simulink model "ad9361_rx_fastattack"  (R2017b)
settings: Solver=ode23  StartTime=0.0  StopTime=inf  RelTol=1e-3  EnableMultiTasking=on
PreLoadFcn:
  | SampleTime_rx = 6.51041666666666667e-8;
  | 
  | adi9361_preload(bdroot,'rx')
undefined symbols (not defined in the file or in its folder): D, dBval, DCLeak_Matrix, fuzz_val, GainImb_Matrix, IP2_Matrix, IP3_Matrix, magnitude, var
libraries: simrfV2elements x13, dsparch4 x8, dspsrcs4 x8, dspmathops x6, dspmlti4 x5, simulink x5, simrfV2util1 x4, fl_lib x4, simrfV2junction1 x3, simulink_extras x2, dspsigattribs x2, simrfV2sources1 x2
(part 2 of 2)

== system ad9361_rx_fastattack/ADI9361_rx/ADC_RX/ADC_Q/Quantizer1 ==
  u : Inport
  Abs : Abs
  Idealized ADC quantizer : simulink_extras/Additional Discrete/Idealized ADC quantizer  NumberOfConverterBits=3  Vmin=0  Vmax=.8  OutputDataType=double  OutputNegativeValues=off
      settings: SourceProductName=Simulink
  Product : Product
  Saturation : Saturate  UpperLimit=0.41
  Sign : Signum
  y : Outport
  wires:
  u/1 -> Sign/1, Abs/1
  Saturation/1 -> Idealized ADC quantizer/1
  Idealized ADC quantizer/1 -> Product/1
  Sign/1 -> Product/2
  Abs/1 -> Saturation/1
  Product/1 -> y/1

== system ad9361_rx_fastattack/ADI9361_rx/DDC_Filters_RX/Hm1/Hm1 ==
  In : Inport
  Hm1 : dspmlti4/FIR Decimation  FilterSource=Filter object  h=fir1(35,0.4)  D=2  filtStruct=Direct form  FilterObject=ad9361_rx_pars.Hm1_rx  framing=Allow multirate processing  inputOffset=0  outputBufInitCond=0  roundingMode=Floor  overflowMode=off  firstCoeffDataTypeStr=Inherit: Same word length as input  firstCoeffMin=[]  firstCoeffMax=[]  firstCoeffLastDataTypeStr=Inherit: Same word length as input  outputDataTypeStr=Inherit: Same as accumulator  outputMin=[]  outputMax=[]  outputLastDataTypeStr=Inherit: Same as accumulator
  Out : Outport
  wires:
  In/1 -> Hm1/1
  Hm1/1 -> Out/1

== system ad9361_rx_fastattack/ADI9361_rx/DDC_Filters_RX/Hm1/NoFilter ==
  In : Inport
  Out : Outport
  wires:
  In/1 -> Out/1

== system ad9361_rx_fastattack/ADI9361_rx/DDC_Filters_RX/Hm2/Hm2 ==
  In : Inport
  Data Type Conversion3 : DataTypeConversion  OutDataTypeStr=fixdt(1,16,14)  RndMeth=Round
  Hm2 : dspmlti4/FIR Decimation  FilterSource=Filter object  h=fir1(35,0.4)  D=2  filtStruct=Direct form  FilterObject=ad9361_rx_pars.Hm2_rx  framing=Allow multirate processing  inputOffset=0  outputBufInitCond=0  roundingMode=Floor  overflowMode=off  firstCoeffDataTypeStr=Inherit: Same word length as input  firstCoeffMin=[]  firstCoeffMax=[]  firstCoeffLastDataTypeStr=Inherit: Same word length as input  outputDataTypeStr=Inherit: Same as accumulator  outputMin=[]  outputMax=[]  outputLastDataTypeStr=Inherit: Same as accumulator
  Out : Outport
  wires:
  In/1 -> Data Type Conversion3/1
  Hm2/1 -> Out/1
  Data Type Conversion3/1 -> Hm2/1

== system ad9361_rx_fastattack/ADI9361_rx/DDC_Filters_RX/Hm2/NoFilter ==
  In : Inport
  Data Type Conversion3 : DataTypeConversion  OutDataTypeStr=fixdt(1,16,14)  RndMeth=Round
  Out : Outport
  wires:
  In/1 -> Data Type Conversion3/1
  Data Type Conversion3/1 -> Out/1

== system ad9361_rx_fastattack/ADI9361_rx/DDC_Filters_RX/Hm3/Hm3 ==
  In : Inport
  Mh3 : dspmlti4/FIR Decimation  FilterSource=Filter object  h=fir1(35,0.4)  D=2  filtStruct=Direct form  FilterObject=ad9361_rx_pars.Hm3_rx  framing=Allow multirate processing  inputOffset=0  outputBufInitCond=0  roundingMode=Floor  overflowMode=off  firstCoeffDataTypeStr=Inherit: Same word length as input  firstCoeffMin=[]  firstCoeffMax=[]  firstCoeffLastDataTypeStr=Inherit: Same word length as input  outputDataTypeStr=Inherit: Same as accumulator  outputMin=[]  outputMax=[]  outputLastDataTypeStr=Inherit: Same as accumulator
  Out : Outport
  wires:
  In/1 -> Mh3/1
  Mh3/1 -> Out/1

== system ad9361_rx_fastattack/ADI9361_rx/DDC_Filters_RX/Hm3/NoFilter ==
  In : Inport
  Out : Outport
  wires:
  In/1 -> Out/1

== system ad9361_rx_fastattack/ADI9361_rx/DDC_Filters_RX/Hm4/Hm4 ==
  In1 : Inport
  Data Type Conversion : DataTypeConversion  OutDataTypeStr=fixdt(1,4,2)  RndMeth=Round
  Hm1 : dspmlti4/FIR Decimation  FilterSource=Filter object  h=fir1(35,0.4)  D=2  filtStruct=Direct form  FilterObject=ad9361_rx_pars.Hm4_rx  framing=Allow multirate processing  inputOffset=0  outputBufInitCond=0  roundingMode=Floor  overflowMode=off  firstCoeffDataTypeStr=Inherit: Same word length as input  firstCoeffMin=[]  firstCoeffMax=[]  firstCoeffLastDataTypeStr=Inherit: Same word length as input  outputDataTypeStr=Inherit: Same as accumulator  outputMin=[]  outputMax=[]  outputLastDataTypeStr=Inherit: Same as accumulator
  Out1 : Outport
  wires:
  In1/1 -> Data Type Conversion/1
  Hm1/1 -> Out1/1
  Data Type Conversion/1 -> Hm1/1

== system ad9361_rx_fastattack/ADI9361_rx/DDC_Filters_RX/Hm4/NoFilter ==
  In1 : Inport
  Data Type Conversion : DataTypeConversion  OutDataTypeStr=fixdt(1,4,2)  RndMeth=Round
  Out1 : Outport
  wires:
  In1/1 -> Data Type Conversion/1
  Data Type Conversion/1 -> Out1/1

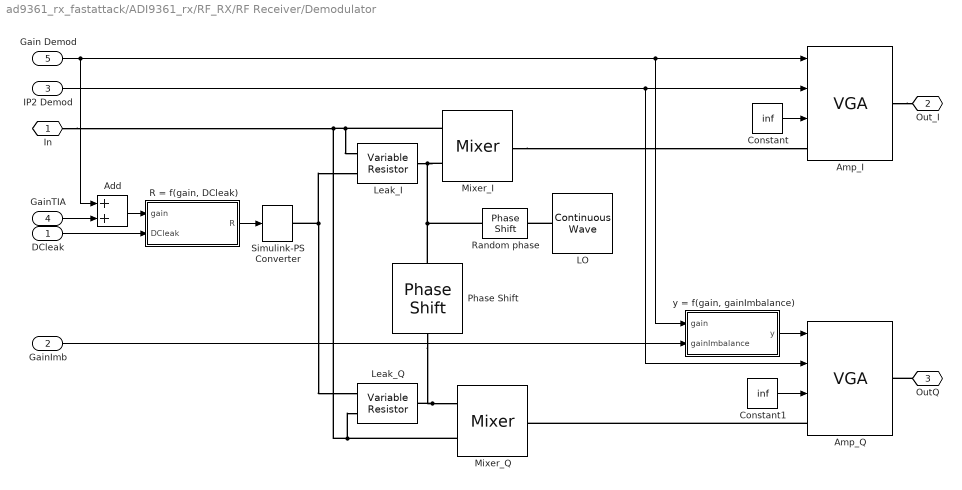
== system ad9361_rx_fastattack/ADI9361_rx/RF_RX/RF Receiver/Demodulator ==
  DCleak : Inport
  GainImb : Inport  Port=2
  IP2 Demod : Inport  Port=3
  GainTIA : Inport  Port=4
  Gain Demod : Inport  Port=5
  Add : Sum
  Amp_I : simrfV2elements/VGA  classname=vga  Zin=100  Zout=100  IO=Input  InternalGrounding=on
      settings: SourceProductName=RF Blockset  SourceProductBaseCode=RB
  Amp_Q : simrfV2elements/VGA  classname=vga  Zin=100  Zout=100  IO=Input  InternalGrounding=on
      settings: SourceProductName=RF Blockset  SourceProductBaseCode=RB
  Constant : Constant  Value=inf
  Constant1 : Constant  Value=inf
  LO : simrfV2sources1/Continuous Wave  CWSourceType=Ideal voltage  Z0=0  IVoltage=1/sqrt(2) V  ICurrent=0 A  MagPower=1 W  QVoltage=0 V  QCurrent=0 A  AnglePower=0  CarrierFreq=RF Hz  InternalGrounding=on
      settings: SourceProductName=RF Blockset  SourceProductBaseCode=RB
  Leak_I : fl_lib/Electrical/Electrical Elements/Variable Resistor  Rmin=0 Ohm  i_specify=off  i_priority=High  i=0 A  v_specify=off  v_priority=High  v=0 V
  Leak_Q : fl_lib/Electrical/Electrical Elements/Variable Resistor  Rmin=0 Ohm  i_specify=off  i_priority=High  i=0 A  v_specify=off  v_priority=High  v=0 V
  Mixer_I : simrfV2elements/Mixer  classname=mixer  Source_linear_gain=Available power gain  linear_gain=0 dB  Zin=100  Zout=100  ZLO=inf  Source_Poly=Even and odd order  Poly_Coeffs=[0 1]  IPType=Output  IP2=Inf dBm  IP3=Inf dBm  P1dB=Inf dBm  Psat=Inf dBm  Gcomp=Inf dBm  NF=0  InternalGrounding=on
      settings: SourceProductName=RF Blockset  SourceProductBaseCode=RB
  Mixer_Q : simrfV2elements/Mixer  classname=mixer  Source_linear_gain=Available power gain  linear_gain=0 dB  Zin=100  Zout=100  ZLO=inf  Source_Poly=Even and odd order  Poly_Coeffs=[0 1]  IPType=Output  IP2=Inf dBm  IP3=Inf dBm  P1dB=Inf dBm  Psat=Inf dBm  Gcomp=Inf dBm  NF=0  InternalGrounding=on
      settings: SourceProductName=RF Blockset  SourceProductBaseCode=RB
  Phase Shift : simrfV2elements/Phase Shift  PhaseShift=90 deg  InternalGrounding=on
      settings: SourceProductName=RF Blockset  SourceProductBaseCode=RB
  "R = f(gain, DCleak)" : Subsystem
  Random phase : simrfV2elements/Phase Shift  PhaseShift=rand(1,1)*360 deg  InternalGrounding=on
      settings: SourceProductName=RF Blockset  SourceProductBaseCode=RB
  Simulink-PS Converter : nesl_utility/Simulink-PS Converter  PhysicalDomain=network_engine_domain  SubClassName=ps_input  LeftPortType=input  RightPortType=output  PseudoPeriodic=off  Frequencies=[]  NoiseDistribution=none  NoiseParameters=[]  Unit=1  AffineConversion=off  InputFiltering=off  SimscapeFilterOrder=1  InputFilterTimeConstant=0.001  UdotUserProvided=1
  "y = f(gain, gainImbalance)" : Subsystem
  In : PMIOPort  Port=1  Side=Left
  Out_I : PMIOPort  Port=2  Side=Right
  OutQ : PMIOPort  Port=3  Side=Right
  wires:
  Gain Demod/1 -> "y = f(gain, gainImbalance)"/1(gain), Amp_I/1, Add/1
  IP2 Demod/1 -> Amp_Q/2, Amp_I/2
  "R = f(gain, DCleak)"/1(R) -> Simulink-PS Converter/1
  GainTIA/1 -> Add/2
  Add/1 -> "R = f(gain, DCleak)"/1(gain)
  GainImb/1 -> "y = f(gain, gainImbalance)"/2(gainImbalance)
  DCleak/1 -> "R = f(gain, DCleak)"/2(DCleak)
  "y = f(gain, gainImbalance)"/1(y) -> Amp_Q/1
  Constant/1 -> Amp_I/3
  Constant1/1 -> Amp_Q/3
  connections:
  Phase Shift/RConn1 -- Mixer_Q/LConn2 -- Leak_Q/RConn1
  Mixer_I/LConn2 -- Random phase/RConn1 -- Phase Shift/LConn1 -- Leak_I/RConn1
  Mixer_Q/LConn1 -- Leak_Q/LConn2 -- In/RConn1 -- Leak_I/LConn2 -- Mixer_I/LConn1
  Amp_I/RConn1 -- Out_I/RConn1
  OutQ/RConn1 -- Amp_Q/RConn1
  Mixer_I/RConn1 -- Amp_I/LConn1
  Amp_Q/LConn1 -- Mixer_Q/RConn1
  Simulink-PS Converter/RConn1 -- Leak_Q/LConn1 -- Leak_I/LConn1
  LO/LConn1 -- Random phase/LConn1

== system ad9361_rx_fastattack/ADI9361_rx/RF_RX/RF Receiver/External LNA ==
  ExternalLNA on/off : Inport
  Bypass : simrfV2junction1/Switch  classname=switch  Ron=0 Ohm  Roff=inf Ohm  Vthres=0.5 V
      settings: SourceProductName=RF Blockset  SourceProductBaseCode=RB
  Invert Control : Subsystem
  LNA : simrfV2elements/Amplifier  classname=amplifier  DataSource=Data file  File=simrfV2_unitygain.s2p  Paramtype=S-parameters  Sparam=[0 0;1 0]  SparamFreq=1e9 Hz  SparamZ0=50  Residues=0  Poles=0  DF={0 0; 1 0}  Source_linear_gain=Available power gain  linear_gain=10 dB  Zin=50  Zout=50  Source_Poly=Even and odd order  Poly_Coeffs=[0 1]  IPType=Output  IP2=inf dBm  IP3=inf dBm  P1dB=inf dBm  Psat=inf dBm  Gcomp=inf dBm  NF=0  InternalGrounding=on  SourceFreq=Extracted from data source  PlotFreq=[1e9:1e6:3e9] Hz  PlotType=X-Y plane  YParam1=S11  YFormat1=Magnitude (decibels)  YParam2=None  YFormat2=Magnitude (decibels)  YOption=Linear  XOption=Linear  SparamRepresentation=Time domain (rationalfit)  FitTol=-40  FitOpt=Fit individually  AutoImpulseLength=on  ImpulseLength=1e-10 s
      settings: SourceProductName=RF Blockset  SourceProductBaseCode=RB
  LNA on input : simrfV2junction1/Switch  classname=switch  Ron=0 Ohm  Roff=inf Ohm  Vthres=0.5 V
      settings: SourceProductName=RF Blockset  SourceProductBaseCode=RB
  LNA on ouput : simrfV2junction1/Switch  classname=switch  Ron=0 Ohm  Roff=inf Ohm  Vthres=0.5 V
      settings: SourceProductName=RF Blockset  SourceProductBaseCode=RB
  in : PMIOPort  Port=1  Side=Left
  out : PMIOPort  Port=2  Side=Right
  wires:
  ExternalLNA on/off/1 -> LNA on ouput/1, LNA on input/1, Invert Control/1(In)
  Invert Control/1(Out) -> Bypass/1
  connections:
  Bypass/RConn1 -- out/RConn1 -- LNA on ouput/RConn1
  LNA on input/LConn1 -- Bypass/LConn1 -- in/RConn1
  LNA on input/RConn1 -- LNA/LConn1
  LNA/RConn1 -- LNA on ouput/LConn1

== system ad9361_rx_fastattack/ADI9361_rx/RF_RX/RF Receiver/RF Non Idealities ==
  LPF : Inport
  TIA : Inport  Port=2
  Demod : Inport  Port=3
  LNA : Inport  Port=4
  DetectChange : Subsystem
  RF Non Idealities : Subsystem
  DCLeakage : Outport
  GainImbalance : Outport  Port=2
  IP2 : Outport  Port=3
  IP3 : Outport  Port=4
  wires:
  TIA/1 -> RF Non Idealities/3(TIA), DetectChange/3(In3)
  LPF/1 -> RF Non Idealities/4(LPF), DetectChange/4(In4)
  Demod/1 -> RF Non Idealities/2(Demod), DetectChange/2(In2)
  LNA/1 -> RF Non Idealities/1(LNA), DetectChange/1(In1)
  RF Non Idealities/1(DCLeakage) -> DCLeakage/1
  RF Non Idealities/2(GainImbalance) -> GainImbalance/1
  RF Non Idealities/3(IP2) -> IP2/1
  RF Non Idealities/4(IP3) -> IP3/1
  DetectChange/1(Trigger) -> RF Non Idealities/Trigger

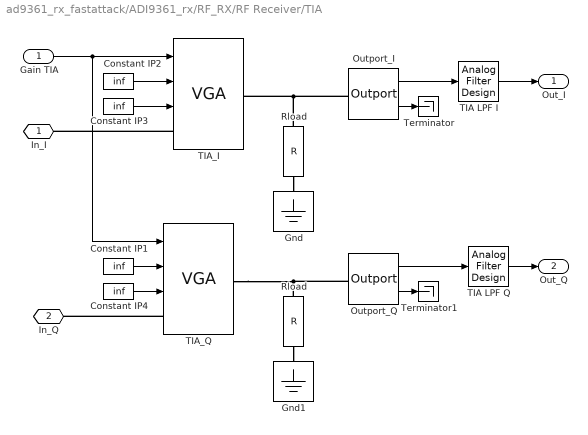
== system ad9361_rx_fastattack/ADI9361_rx/RF_RX/RF Receiver/TIA ==
  Gain TIA : Inport
  " Rload" : simrfV2elements/R  classname=resistor  Resistance=100 Ohm  AddNoise=on
      settings: SourceProductName=RF Blockset  SourceProductBaseCode=RB
  Constant IP{1..4} (4 alike) : Constant  Value=inf
  Gnd : fl_lib/Electrical/Electrical Elements/Electrical Reference
  Gnd1 : fl_lib/Electrical/Electrical Elements/Electrical Reference
  Outport_I : simrfV2util1/Outport  SensorType=Ideal voltage  OutputFormat=In-phase and Quadrature Baseband  CarrierFreq=0 Hz  ZL=Inf  InternalGrounding=on  StepSize=-1 s  AutoStep=off
      settings: SourceProductName=RF Blockset  SourceProductBaseCode=RB
  Outport_Q : simrfV2util1/Outport  SensorType=Ideal voltage  OutputFormat=In-phase and Quadrature Baseband  CarrierFreq=0 Hz  ZL=Inf  InternalGrounding=on  StepSize=-1 s  AutoStep=off
      settings: SourceProductName=RF Blockset  SourceProductBaseCode=RB
  Rload : simrfV2elements/R  classname=resistor  Resistance=100 Ohm  AddNoise=on
      settings: SourceProductName=RF Blockset  SourceProductBaseCode=RB
  TIA LPF I : dsparch4/Analog Filter Design  method=Butterworth  filttype=Lowpass  N=1  Wlo=2.5*ad9361_rx_pars.Fpass*2*pi  Whi=80  Rp=2  Rs=40
  TIA LPF Q : dsparch4/Analog Filter Design  method=Butterworth  filttype=Lowpass  N=1  Wlo=2.5*ad9361_rx_pars.Fpass*2*pi  Whi=80  Rp=2  Rs=40
  TIA_I : simrfV2elements/VGA  classname=vga  Zin=100  Zout=100  IO=Input  InternalGrounding=on
      settings: SourceProductName=RF Blockset  SourceProductBaseCode=RB
  TIA_Q : simrfV2elements/VGA  classname=vga  Zin=100  Zout=100  IO=Input  InternalGrounding=on
      settings: SourceProductName=RF Blockset  SourceProductBaseCode=RB
  Terminator : Terminator
  Terminator1 : Terminator
  In_I : PMIOPort  Port=1  Side=Left
  In_Q : PMIOPort  Port=2  Side=Left
  Out_I : Outport
  Out_Q : Outport  Port=2
  wires:
  Outport_Q/1 -> TIA LPF Q/1
  Outport_I/1 -> TIA LPF I/1
  Outport_I/2 -> Terminator/1
  Outport_Q/2 -> Terminator1/1
  Gain TIA/1 -> TIA_Q/1, TIA_I/1
  TIA LPF I/1 -> Out_I/1
  TIA LPF Q/1 -> Out_Q/1
  Constant IP2/1 -> TIA_I/2
  Constant IP3/1 -> TIA_I/3
  Constant IP1/1 -> TIA_Q/2
  Constant IP4/1 -> TIA_Q/3
  connections:
  TIA_I/LConn1 -- In_I/RConn1
  TIA_Q/LConn1 -- In_Q/RConn1
  Outport_I/LConn1 -- Rload/LConn1 -- TIA_I/RConn1
  Outport_Q/LConn1 -- TIA_Q/RConn1 -- " Rload"/LConn1
  Rload/RConn1 -- Gnd/LConn1
  " Rload"/RConn1 -- Gnd1/LConn1

== system ad9361_rx_fastattack/ADI9361_rx/RF_RX/RF Receiver/Demodulator/R = f(gain, DCleak) ==
  gain : Inport
  DCleak : Inport  Port=2
  Add : Sum  Inputs=--+-+
  Add1 : Sum  Inputs=+-
  Constant1 : Constant  Value=20
  Constant2 : Constant  Value=27
  Constant3 : Constant  Value=3
  Constant4 : Constant  Value=25
  Gain1 : Gain  Gain=(-1)/20
  Gain2 : Gain  Gain=25
  expon3 : Math  Operator=10^u  SaturateOnIntegerOverflow=on
  R : Outport
  wires:
  Add1/1 -> R/1
  Constant4/1 -> Add1/2
  Gain2/1 -> Add1/1
  Gain1/1 -> expon3/1
  Constant2/1 -> Add/4
  Constant1/1 -> Add/3
  Constant3/1 -> Add/2
  DCleak/1 -> Add/5
  Add/1 -> Gain1/1
  gain/1 -> Add/1
  expon3/1 -> Gain2/1

== system ad9361_rx_fastattack/ADI9361_rx/RF_RX/RF Receiver/Demodulator/y = f(gain, gainImbalance) ==
  gain : Inport
  gainImbalance : Inport  Port=2
  Add2 : Sum
  Constant2 : Constant  Value=2
  Gain4 : Gain  Gain=1/20
  Gain5 : Gain  Gain=1/20
  Gain6 : Gain  Gain=20
  Times1 : Product  Inputs=***
  expon2 : Math  Operator=10^u  SaturateOnIntegerOverflow=on
  expon3 : Math  Operator=10^u  SaturateOnIntegerOverflow=on
  log1 : Math  Operator=log10  SaturateOnIntegerOverflow=on
  y : Outport
  wires:
  expon2/1 -> Times1/2
  Gain5/1 -> expon3/1
  Times1/1 -> Add2/2
  Gain4/1 -> expon2/1
  Add2/1 -> log1/1
  log1/1 -> Gain6/1
  gain/1 -> Gain5/1
  expon3/1 -> Times1/1, Add2/1
  gainImbalance/1 -> Gain4/1
  Constant2/1 -> Times1/3
  Gain6/1 -> y/1

== system ad9361_rx_fastattack/ADI9361_rx/RF_RX/RF Receiver/External LNA/Invert Control ==
  In : Inport
  Data Type Conversion : DataTypeConversion  OutDataTypeStr=boolean
  Data Type Conversion1 : DataTypeConversion  OutDataTypeStr=double
  Logical Operator : Logic  Operator=NOT  AllPortsSameDT=off  OutDataTypeStr=boolean
  Out : Outport
  wires:
  In/1 -> Data Type Conversion/1
  Logical Operator/1 -> Data Type Conversion1/1
  Data Type Conversion/1 -> Logical Operator/1
  Data Type Conversion1/1 -> Out/1

== system ad9361_rx_fastattack/ADI9361_rx/RF_RX/RF Receiver/RF Non Idealities/DetectChange ==
  In1 : Inport
  In2 : Inport  Port=2
  In3 : Inport  Port=3
  In4 : Inport  Port=4
  Detect Change{,1..4} (5 alike) : simulink/Logic and Bit Operations/Detect Change  vinit=0  InputProcessing=Inherited  OutDataTypeStr=boolean
  Logical Operator : Logic  Operator=OR  Inputs=5  AllPortsSameDT=off  OutDataTypeStr=boolean
  Step : Step  Time=2*Tstep  SampleTime=Tstep  VectorParams1D=off  ZeroCross=off
  Trigger : Outport
  wires:
  Detect Change/1 -> Logical Operator/4
  Detect Change1/1 -> Logical Operator/3
  Detect Change2/1 -> Logical Operator/2
  In4/1 -> Detect Change3/1
  In2/1 -> Detect Change1/1
  In3/1 -> Detect Change2/1
  Detect Change3/1 -> Logical Operator/1
  In1/1 -> Detect Change/1
  Logical Operator/1 -> Trigger/1
  Detect Change4/1 -> Logical Operator/5
  Step/1 -> Detect Change4/1

== system ad9361_rx_fastattack/ADI9361_rx/RF_RX/RF Receiver/RF Non Idealities/RF Non Idealities ==
  LNA : Inport
  Demod : Inport  Port=2
  TIA : Inport  Port=3
  LPF : Inport  Port=4
  Trigger : TriggerPort  VariantControl=Variant  PortDimensions=1
  RF NonIdealities : MATLAB Function  TreatAsAtomicUnit=on
      mask init:
      | load ADI9361Tables;
  DCLeakage : Outport
  GainImbalance : Outport  Port=2
  IP2 : Outport  Port=3
  IP3 : Outport  Port=4
  wires:
  RF NonIdealities/1(Leak) -> DCLeakage/1
  RF NonIdealities/2(GainImb) -> GainImbalance/1
  RF NonIdealities/3(IP2) -> IP2/1
  RF NonIdealities/4(IP3) -> IP3/1
  LNA/1 -> RF NonIdealities/1(LNA)
  LPF/1 -> RF NonIdealities/4(LPF)
  Demod/1 -> RF NonIdealities/2(Demod)
  TIA/1 -> RF NonIdealities/3(TIA)

== matlab function ad9361_rx_fastattack/ADI9361_rx/RF_RX/RF Receiver/RF Non Idealities/RF Non Idealities/RF NonIdealities ==
  data: LNA input; Leak output; Demod input; TIA input; LPF input; GainImb output; IP2 output; IP3 output; DCLeak_Matrix parameter; GainImb_Matrix parameter; IP3_Matrix parameter; IP2_Matrix parameter
function [Leak, GainImb, IP2, IP3] =                                    ...
    nonIdealsRF(LNA, Demod, TIA, LPF, DCLeak_Matrix, GainImb_Matrix,    ...
    IP3_Matrix, IP2_Matrix)
%#codegen
coder.extrinsic('griddatan','warning');
IP2 = 200;
IP3 = 200;
Leak = -200;
GainImb = -200;
Leak(:) = griddatan(DCLeak_Matrix(:,1:4), DCLeak_Matrix(:,5),           ...
    [LNA, Demod, TIA, LPF]);
GainImb(:) = griddatan(GainImb_Matrix(:,1:4), GainImb_Matrix(:,5),      ...
    [LNA, Demod, TIA, LPF]);
IP2(:) = griddatan(IP2_Matrix(:,1:4), IP2_Matrix(:,5),[LNA,Demod,TIA,LPF]);
IP3(:) = griddatan(IP3_Matrix(:,1:4), IP3_Matrix(:,5),[LNA,Demod,TIA,LPF]);

if isnan(IP2)
    IP2(:) = griddatan(IP2_Matrix(:,1:4), IP2_Matrix(:,5),              ...
        [LNA, Demod, TIA, LPF],'nearest');
    % Warning('Failed interpolation on IP2');
end
if isnan(IP3)
    IP3(:) = griddatan(IP3_Matrix(:,1:4), IP3_Matrix(:,5),              ...
        [LNA, Demod, TIA, LPF],'nearest');
    % Warning('Failed interpolation on IP3');
end
if isnan(Leak)
    Leak(:) = griddatan(DCLeak_Matrix(:,1:4), DCLeak_Matrix(:,5),       ...
        [LNA, Demod, TIA, LPF],'nearest');
    % Warning('Failed interpolation on DC leakage');
end
if isnan(GainImb)
    GainImb(:) = griddatan(GainImb_Matrix(:,1:4), GainImb_Matrix(:,5),  ...
        [LNA, Demod, TIA, LPF],'nearest');
    % Warning('Failed interpolation on Gain Imbalance');
end

IP2 = 2*(IP2+LNA);

== stateflow chart ad9361_rx_fastattack/ADI9361_rx/AGC ==
  settings: executeAtInitialization=1
  state InitialState
    gain_index=76;
  state AGC_SEL
  state SlowAttackMode
    state CheckOverloads
    state ResetLMTMeter
    state ResetADCMeter
    state ResetPMeter1
    state ResetPMeter2
    state ResetPMeter3
    state ResetPMeter4
    state DECREASE_GAIN_Inner
      entry:
      gain_index = max(gain_index-AGC_G_dec_slow,0);
    state INCREASE_GAIN_Inner
      entry:
      gain_index = min(gain_index+AGC_G_inc_slow,76);
    state DECREASE_GAIN_Outer
      entry:
      gain_index = max(gain_index-AGC_G_dec_fast,0);
    state INCREASE_GAIN_Outer
      entry:
      gain_index = min(gain_index+AGC_G_inc_fast,76);
    state DECREASE_GAIN_ADC
      exit:
      gain_index = max(gain_index-ADC_G_dec_fast,0);
    state DECREASE_GAIN_LMT
      exit:
      gain_index = max(gain_index-LMT_G_dec_fast,0);
    (default) -> CheckOverloads
    ResetLMTMeter -> CheckOverloads : after(PeakOverLoadWait,sec)
    CheckOverloads -> DECREASE_GAIN_LMT [order 1] : at(N_LMT_H, LMT_H)
    ResetADCMeter -> CheckOverloads : after(PeakOverLoadWait,sec)
    CheckOverloads -> DECREASE_GAIN_ADC [order 2] : at(N_ADC_H, ADC_H)
    ResetPMeter1 -> CheckOverloads : after(SettlingDelay,sec)
    CheckOverloads -> DECREASE_GAIN_Outer [order 3] : [after(C,sec)&&avg_power>PT_HH]
    ResetPMeter2 -> CheckOverloads : after(SettlingDelay,sec)
    CheckOverloads -> DECREASE_GAIN_Inner [order 4] : [after(C,sec)&&avg_power>PT_H]
    ResetPMeter3 -> CheckOverloads : after(SettlingDelay,sec)
    CheckOverloads -> INCREASE_GAIN_Outer [order 5] : [after(C,sec)&&avg_power<PT_LL]
    ResetPMeter4 -> CheckOverloads : after(SettlingDelay,sec)
    CheckOverloads -> INCREASE_GAIN_Inner [order 6] : [after(C,sec)&&avg_power<PT_L]
    DECREASE_GAIN_ADC -> ResetADCMeter : after(C,sec)
    DECREASE_GAIN_Outer -> ResetPMeter1
    DECREASE_GAIN_Inner -> ResetPMeter2
    INCREASE_GAIN_Outer -> ResetPMeter3
    INCREASE_GAIN_Inner -> ResetPMeter4
    DECREASE_GAIN_LMT -> ResetLMTMeter : after(C,sec)
  state ManualGainControl
    state DoNothing
    state CHANGE_GAIN
      entry:
      gain_index = ManualGainIndex;
    (default) -> DoNothing
    CHANGE_GAIN -> DoNothing : after(1e-6,sec)
    DoNothing -> (junction 345) : after(1e-6,sec)
    (junction 345) -> CHANGE_GAIN : [ManualGainIndex>0 && ManualGainIndex<77]
  state FastAttackMode
    state State0
    state DecreaseGainFast
      entry:
      gain_index =max(gain_index-AGC_G_dec_fast,0);
    state State1
      entry:
      Lock = 0;
      count = 0;
    state DecreaseGainSlow
      entry:
      gain_index =max(gain_index-AGC_G_dec_slow,0);
    state Wait
    state State2_measLP
      entry:
      LP = 1;
      during:
      LP = (avg_power<LowPower)*LP;
    state State2A
      entry:
      LP = 1;
      during:
      LP = (avg_power<LowPower)*LP;
    state IncreaseGain
      entry:
      gain_index = min(gain_index+AGC_G_inc_fast,76);
    state ResetPM [commented out]
    state State2_setGain
      entry:
      gain_change = min(int8(AGC_lock_level-avg_power), Max_Increase)
      gain_index = min(max(gain_index+gain_change, 0),76)
      gain_begin = gain_index;
    state State3
      entry:
      LP = 1;
      during:
      LP = (avg_power<LowPower)*LP;
    state State4
      entry:
      count = count+1;
      gain_index =max(gain_index-PostLockStepSize,0);
    state State5_measPow
      entry:
      Lock = 1;
      count = 0;
      exit:
      init_power = avg_power;
    state ResetGain
      ResetGain -> (junction 449) [order 1]
      (junction 450) -> ResetGain
      (junction 449) -> (junction 450) [order 1] : [GainReset==1]/{gain_index=76}
      (junction 449) -> (junction 454) [order 2]
      (junction 458) -> ResetGain
      (junction 454) -> (junction 458) [order 2] : [GainReset==2]/{gain_index=min(max(gain_end+GainOffset, 0),76) }
      (junction 454) -> (junction 456) [order 1]
      (junction 460) -> ResetGain
      (junction 456) -> (junction 460) [order 1] : [GainReset==3]/{gain_index=gain_begin}
      (junction 456) -> ResetGain [order 2] : [GainReset==4]
    state PowerMeas_5
      entry:
      PA =avg_power;
      exit:
      gain_end = gain_index;
    state Counter
      entry:
      count = count+1;
    (default) -> State0
    State0 -> State1 : after(AGC_attack_delay*1e-6,sec)
    State2_measLP -> DecreaseGainFast [order 1] : [at(1,LMT_H) || at(1,ADC_H)]
    State1 -> DecreaseGainFast [order 1] : [at(1,LMT_H) || at(1,ADC_H)]
    DecreaseGainFast -> State1 : after(PeakOverLoadWait,sec)
    State2_measLP -> DecreaseGainSlow [order 2] : at(1,ADC_L)
    ResetPM -> State1 [commented out] : after(DecPowerMeasDuration, sec)
    State1 -> DecreaseGainSlow [order 2] : at(1,ADC_L)
    (junction 466) -> State1
    DecreaseGainSlow -> State1 : after(PeakOverLoadWait,sec)
    (junction 422) -> State1 [order 2]
    State1 -> Wait [order 3] : after(EnergyDetectCount,sec)
    Wait -> State2_measLP : [after(max(SettlingDelay-EnergyDetectCount,0),sec)]
    State2A -> (junction 422) : after(IncrTime, sec)
    (junction 422) -> IncreaseGain [order 1] : [LP && EnableIncrGain]
    IncreaseGain -> State2A : after(DecPowerMeasDuration, sec)
    (junction 428) -> State2A [order 1] : [LP && EnableIncrGain && EnableGainIncAfterLock]/{Lock=0}
    (junction 407) -> State2A [order 1] : [LP && EnableIncrGain]
    State2_measLP -> (junction 407) [order 3] : after(DecPowerMeasDuration, sec)
    (junction 407) -> State2_setGain [order 2]
    State2_setGain -> State3 : {Lock=1}
    State3 -> State4 [order 1] : [at(1,LMT_H) || at(1,ADC_H)]/{Lock = 0}
    State4 -> (junction 466) [order 1] : [count>Overrange]
    ResetGain -> (junction 466) [order 1]
    (junction 463) -> (junction 466)
    State4 -> State3 [order 2]
    State3 -> (junction 428) [order 2] : after(DecPowerMeasDuration, sec)
    (junction 428) -> State5_measPow [order 2]
    State5_measPow -> PowerMeas_5 : [after(PowerMeasDuration,sec)]
    (junction 436) -> ResetGain [order 1] : [count>2*GainLockExitCount]/{Lock=0}
    (junction 436) -> PowerMeas_5 [order 2] : [after(FIR_Ts,sec)]
    Counter -> (junction 436)
    PowerMeas_5 -> PowerMeas_5 [order 2] : [after(PowerMeasDuration,sec)]
    PowerMeas_5 -> Counter [order 4] : [(init_power-PA)>EnergyLost]
    PowerMeas_5 -> (junction 463) [order 1] : [at(1,LMT_H) || at(1,ADC_H)]/{Lock=0}
    PowerMeas_5 -> (junction 463) [order 3] : [(PA-init_power)>StrongerSignalThreshold]
  (default) -> InitialState
  InitialState -> AGC_SEL : after(T*1e-6,sec)
  FastAttackMode -> AGC_SEL : [mode!=2]
  AGC_SEL -> SlowAttackMode [order 3] : [mode==0]
  SlowAttackMode -> AGC_SEL : [mode!=0]
  AGC_SEL -> FastAttackMode [order 2] : [mode==2]
  AGC_SEL -> ManualGainControl [order 1] : [mode==1]
  ManualGainControl -> AGC_SEL : [mode!=1]
  data: mode input; N_LMT_H parameter double; N_ADC_H parameter double; C parameter; ADC_G_dec_fast parameter; AGC_G_inc_fast parameter; AGC_G_inc_slow parameter; LMT_G_dec_fast parameter; AGC_G_dec_fast parameter; AGC_G_dec_slow parameter; avg_power input; ManualGainIndex parameter double; AGC_attack_delay parameter double; EnergyDetectCount parameter double; EnableIncrGain parameter double; IncrTime parameter; FIR_Ts parameter; T parameter; AGC_lock_level parameter double; EnableGainIncAfterLock parameter; Max_Increase parameter; gain_change local double; Overrange parameter; PostLockStepSize parameter; count local double; Lock local double; EnergyLost parameter; GainLockExitCount parameter; init_power local double; LowPower parameter; PowerMeasDuration parameter; LP local double; PA local double; PeakOverLoadWait parameter; GainOffset parameter; StrongerSignalThreshold parameter; gain_begin local double; GainReset parameter; PT_H parameter; PT_HH parameter; PT_L parameter; PT_LL parameter; SettlingDelay parameter; gain_index output double; DecPowerMeasDuration parameter; gain_end local double
  events: ADC_H input EITHER_EDGE_EVENT; ADC_L input EITHER_EDGE_EVENT; LMT_L input EITHER_EDGE_EVENT; LMT_H input EITHER_EDGE_EVENT; event input EITHER_EDGE_EVENT
